simulink model "main_system312XY"  (R2020a)
settings: Solver=daessc  StartTime=0.0  StopTime=10  RelTol=1e-3
model workspace (MAT data in the model file):
  Vmax : Simulink.Parameter (value not decoded)
values from neighbouring files (symbols this model uses):
  motor_diamter = 25/1000    (= 0.025)    [parameters.m]
  motor_height = 56/1000    (= 0.056)    [parameters.m]
  pulley_diameterOut = 1/100    (= 0.01)    [parameters.m]
undefined symbols (not defined in the file or in its folder): Local, sigbuilder_block, X, Y, Z
libraries: sm_lib x59, Multibody_Parts_Lib x22, nesl_utility x7, simulink x3
(part 2 of 2)

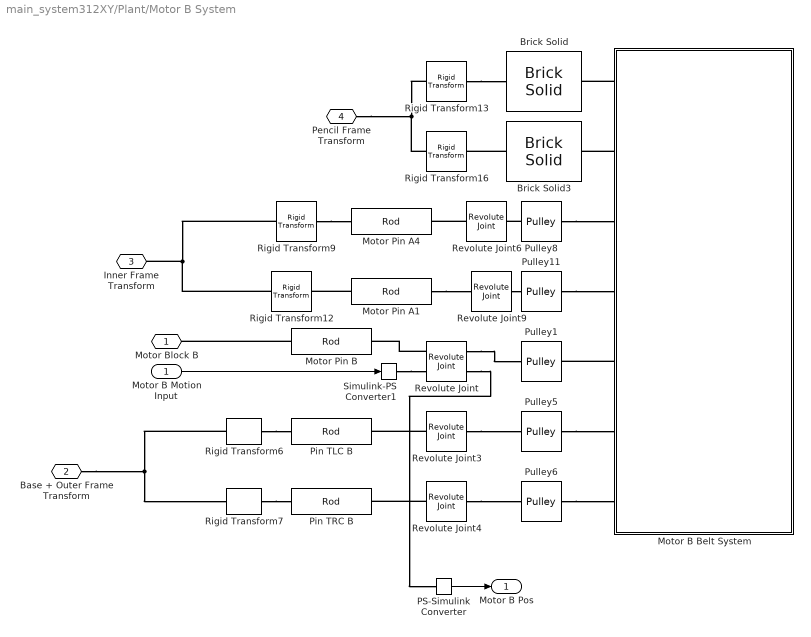
== system main_system312XY/Plant/Motor B System ==
  Motor B Motion Input : Inport
  Brick Solid : sm_lib/Body Elements/Brick Solid  GraphicAmbientColor=[0.15 0.15 0.15 1.0]  BasedOnType=Density  BrickDimensions=end_stop_size  BrickDimensionUnits=cm  CenterOfMass=[0 0 0]  CenterOfMassUnits=m  GraphicDiffuseColor=[0.5 0.5 0.5]  Density=1000  DensityUnits=kg/m^3  DoExposeReferenceFrame=on  GraphicEmissiveColor=[0.0 0.0 0.0 1.0]  ExportEntireGeometry=off  SerializedFrames=<Frames><Frame><Id>Frame1</Id><Value><Name>Bottom</Name><Origin><Source>GeometricFeature</Source><FeatureName>-z surface</FeatureName></Origin><PrimaryAxis><DefinedDirection>+Z</DefinedDirection><Source>ReferenceFrame</Source><SourceDirection>+Z</SourceDirection><FeatureName></FeatureName></PrimaryAxis><SecondaryAxis><DefinedDirection>+X</DefinedDirection><Source>ReferenceFrame</Source><SourceDirection>+X</SourceDirection><FeatureName></FeatureName></SecondaryAxis></Value></Frame></Frames>  MarkerShape=Sphere  MarkerSize=10  GraphicType=FromGeometry  InertiaType=CalculateFromGeometry  Mass=1  MassUnits=kg  MomentsOfInertia=[1 1 1]  MomentsOfInertiaUnits=kg*m^2  GraphicOpacity=1.0  ProductsOfInertia=[0 0 0]  ProductsOfInertiaUnits=kg*m^2  GraphicShininess=75  GraphicSpecularColor=[0.5 0.5 0.5 1.0]  GraphicVisPropType=SimpleVisualProperties
  Brick Solid3 : sm_lib/Body Elements/Brick Solid  GraphicAmbientColor=[0.15 0.15 0.15 1.0]  BasedOnType=Density  BrickDimensions=end_stop_size  BrickDimensionUnits=cm  CenterOfMass=[0 0 0]  CenterOfMassUnits=m  GraphicDiffuseColor=[0.5 0.5 0.5]  Density=1000  DensityUnits=kg/m^3  DoExposeReferenceFrame=on  GraphicEmissiveColor=[0.0 0.0 0.0 1.0]  ExportEntireGeometry=off  SerializedFrames=<Frames><Frame><Id>Frame1</Id><Value><Name>Bottom</Name><Origin><Source>GeometricFeature</Source><FeatureName>-z surface</FeatureName></Origin><PrimaryAxis><DefinedDirection>+Z</DefinedDirection><Source>ReferenceFrame</Source><SourceDirection>+Z</SourceDirection><FeatureName></FeatureName></PrimaryAxis><SecondaryAxis><DefinedDirection>+X</DefinedDirection><Source>ReferenceFrame</Source><SourceDirection>+X</SourceDirection><FeatureName></FeatureName></SecondaryAxis></Value></Frame></Frames>  MarkerShape=Sphere  MarkerSize=10  GraphicType=FromGeometry  InertiaType=CalculateFromGeometry  Mass=1  MassUnits=kg  MomentsOfInertia=[1 1 1]  MomentsOfInertiaUnits=kg*m^2  GraphicOpacity=1.0  ProductsOfInertia=[0 0 0]  ProductsOfInertiaUnits=kg*m^2  GraphicShininess=75  GraphicSpecularColor=[0.5 0.5 0.5 1.0]  GraphicVisPropType=SimpleVisualProperties
  Motor B Belt System : Subsystem
  Motor Pin A1 : Multibody_Parts_Lib/Basic/Rod  rod_rad=pulley_diameterInner  rod_len=pulley_pin_height  rod_rho=7000  rod_color=motor_colA  rod_opc=1  popup_zori=Local +Z  popup_markings=None  mark_radius_range=[0.5 1.01]  mark_length_range=1.005  mark_angle_range=30  mark_color=[1 1 1]
      settings: SourceProductName=Simscape Multibody Parts Library
  Motor Pin A4 : Multibody_Parts_Lib/Basic/Rod  rod_rad=pulley_diameterInner  rod_len=pulley_pin_height  rod_rho=7000  rod_color=motor_colA  rod_opc=1  popup_zori=Local +Z  popup_markings=None  mark_radius_range=[0.5 1.01]  mark_length_range=1.005  mark_angle_range=30  mark_color=[1 1 1]
      settings: SourceProductName=Simscape Multibody Parts Library
  Motor Pin B : Multibody_Parts_Lib/Basic/Rod  rod_rad=pulley_diameterInner  rod_len=pulley_pin_height  rod_rho=7000  rod_color=motor_colB  rod_opc=1  popup_zori=Local +Z  popup_markings=None  mark_radius_range=[0.5 1.01]  mark_length_range=1.005  mark_angle_range=30  mark_color=[1 1 1]
      settings: SourceProductName=Simscape Multibody Parts Library
  PS-Simulink Converter : nesl_utility/PS-Simulink Converter  PhysicalDomain=network_engine_domain  SubClassName=ps_output  LeftPortType=input  RightPortType=output  PseudoPeriodic=off  Frequencies=[]  Unit=inherit  AffineConversion=off
  Pin TLC B : Multibody_Parts_Lib/Basic/Rod  rod_rad=pulley_diameterInner  rod_len=pulley_pin_height  rod_rho=7000  rod_color=motor_colA  rod_opc=1  popup_zori=Local +Z  popup_markings=None  mark_radius_range=[0.5 1.01]  mark_length_range=1.005  mark_angle_range=30  mark_color=[1 1 1]
      settings: SourceProductName=Simscape Multibody Parts Library
  Pin TRC B : Multibody_Parts_Lib/Basic/Rod  rod_rad=pulley_diameterInner  rod_len=pulley_pin_height  rod_rho=7000  rod_color=motor_colA  rod_opc=1  popup_zori=Local +Z  popup_markings=None  mark_radius_range=[0.5 1.01]  mark_length_range=1.005  mark_angle_range=30  mark_color=[1 1 1]
      settings: SourceProductName=Simscape Multibody Parts Library
  Pulley1 : Multibody_Parts_Lib/Basic/Pulley  pulley_rad=pulley_diameterOut/2  pulley_d_grv=pulley_diameterOut/2  pulley_a_grv=45  pulley_th=pulley_height  pulley_radh=0.005  pulley_rho=7000  pulley_clr=[0.6 0.6 0.6]  pulley_opc=1  pulley_zori=No  popup_markings=Two  mark_radius_range=[0.7 0.9]  mark_angle_range=60  mark_color=[1 1 1]
      settings: SourceProductName=Simscape Multibody Parts Library
  Pulley11 : Multibody_Parts_Lib/Basic/Pulley  pulley_rad=pulley_diameterOut/2  pulley_d_grv=pulley_diameterOut/2  pulley_a_grv=45  pulley_th=0.01  pulley_radh=0.005  pulley_rho=7000  pulley_clr=[0.6 0.6 0.6]  pulley_opc=1  pulley_zori=No  popup_markings=Two  mark_radius_range=[0.7 0.9]  mark_angle_range=60  mark_color=[1 1 1]
      settings: SourceProductName=Simscape Multibody Parts Library
  Pulley5 : Multibody_Parts_Lib/Basic/Pulley  pulley_rad=pulley_diameterOut/2  pulley_d_grv=pulley_diameterOut/2  pulley_a_grv=45  pulley_th=pulley_height  pulley_radh=0.005  pulley_rho=7000  pulley_clr=[0.6 0.6 0.6]  pulley_opc=1  pulley_zori=No  popup_markings=Two  mark_radius_range=[0.7 0.9]  mark_angle_range=60  mark_color=[1 1 1]
      settings: SourceProductName=Simscape Multibody Parts Library
  Pulley6 : Multibody_Parts_Lib/Basic/Pulley  pulley_rad=pulley_diameterOut/2  pulley_d_grv=pulley_diameterOut/2  pulley_a_grv=45  pulley_th=pulley_height  pulley_radh=0.005  pulley_rho=7000  pulley_clr=[0.6 0.6 0.6]  pulley_opc=1  pulley_zori=No  popup_markings=Two  mark_radius_range=[0.7 0.9]  mark_angle_range=60  mark_color=[1 1 1]
      settings: SourceProductName=Simscape Multibody Parts Library
  Pulley8 : Multibody_Parts_Lib/Basic/Pulley  pulley_rad=pulley_diameterOut/2  pulley_d_grv=pulley_diameterOut/2  pulley_a_grv=45  pulley_th=0.01  pulley_radh=0.005  pulley_rho=7000  pulley_clr=[0.6 0.6 0.6]  pulley_opc=1  pulley_zori=No  popup_markings=Two  mark_radius_range=[0.7 0.9]  mark_angle_range=60  mark_color=[1 1 1]
      settings: SourceProductName=Simscape Multibody Parts Library
  Revolute Joint : sm_lib/Joints/Revolute Joint  JointMode=Normal  SenseConstraintForce=off  SenseConstraintForceX=off  SenseConstraintForceY=off  SenseConstraintForceZ=off  SenseConstraintTorque=off  SenseConstraintTorqueX=off  SenseConstraintTorqueY=off  SenseConstraintTorqueZ=off  SenseTotalForce=off  SenseTotalForceX=off  SenseTotalForceY=off  SenseTotalForceZ=off  SenseTotalTorque=off  SenseTotalTorqueX=off  SenseTotalTorqueY=off  SenseTotalTorqueZ=off  CompositeWrenchDir=FollowerOnBase  CompositeWrenchFrame=BaseFrame  EquilibriumPosition=0  EquilibriumPositionUnits=deg  SpringStiffness=0  SpringStiffnessUnits=N*m/deg  DampingCoefficient=0  DampingCoefficientUnits=N*m/(deg/s)  TorqueActuationMode=ComputedTorque  MotionActuationMode=InputMotion  SensePosition=on  SenseVelocity=off  SenseAcceleration=off  SenseTorqueForce=off  SenseLowerLimitTorqueForce=off  SenseUpperLimitTorqueForce=off  LowerLimitSpecify=off  LowerLimitBound=-90  LowerLimitBoundUnits=deg  LowerLimitStiffness=1e4  LowerLimitStiffnessUnits=N*m/deg  LowerLimitDamping=10  LowerLimitDampingUnits=N*m/(deg/s)  LowerLimitTransitionRegionWidth=0.1  LowerLimitTransitionRegionWidthUnits=deg  UpperLimitSpecify=off  UpperLimitBound=90  UpperLimitBoundUnits=deg  UpperLimitStiffness=1e4  UpperLimitStiffnessUnits=N*m/deg  UpperLimitDamping=10  UpperLimitDampingUnits=N*m/(deg/s)  UpperLimitTransitionRegionWidth=0.1  UpperLimitTransitionRegionWidthUnits=deg  PositionTargetSpecify=off  PositionTargetPriority=High  PositionTargetValue=0  PositionTargetValueUnits=deg  VelocityTargetSpecify=off  VelocityTargetPriority=High  VelocityTargetValue=0  VelocityTargetValueUnits=deg/s
  Revolute Joint{3..4,6,9} (4 alike) : sm_lib/Joints/Revolute Joint  JointMode=Normal  SenseConstraintForce=off  SenseConstraintForceX=off  SenseConstraintForceY=off  SenseConstraintForceZ=off  SenseConstraintTorque=off  SenseConstraintTorqueX=off  SenseConstraintTorqueY=off  SenseConstraintTorqueZ=off  SenseTotalForce=off  SenseTotalForceX=off  SenseTotalForceY=off  SenseTotalForceZ=off  SenseTotalTorque=off  SenseTotalTorqueX=off  SenseTotalTorqueY=off  SenseTotalTorqueZ=off  CompositeWrenchDir=FollowerOnBase  CompositeWrenchFrame=BaseFrame  EquilibriumPosition=0  EquilibriumPositionUnits=deg  SpringStiffness=0  SpringStiffnessUnits=N*m/deg  DampingCoefficient=0  DampingCoefficientUnits=N*m/(deg/s)  TorqueActuationMode=NoTorque  MotionActuationMode=ComputedMotion  SensePosition=off  SenseVelocity=off  SenseAcceleration=off  SenseTorqueForce=off  SenseLowerLimitTorqueForce=off  SenseUpperLimitTorqueForce=off  LowerLimitSpecify=off  LowerLimitBound=-90  LowerLimitBoundUnits=deg  LowerLimitStiffness=1e4  LowerLimitStiffnessUnits=N*m/deg  LowerLimitDamping=10  LowerLimitDampingUnits=N*m/(deg/s)  LowerLimitTransitionRegionWidth=0.1  LowerLimitTransitionRegionWidthUnits=deg  UpperLimitSpecify=off  UpperLimitBound=90  UpperLimitBoundUnits=deg  UpperLimitStiffness=1e4  UpperLimitStiffnessUnits=N*m/deg  UpperLimitDamping=10  UpperLimitDampingUnits=N*m/(deg/s)  UpperLimitTransitionRegionWidth=0.1  UpperLimitTransitionRegionWidthUnits=deg  PositionTargetSpecify=off  PositionTargetPriority=High  PositionTargetValue=0  PositionTargetValueUnits=deg  VelocityTargetSpecify=off  VelocityTargetPriority=High  VelocityTargetValue=0  VelocityTargetValueUnits=deg/s
  Rigid Transform12 : sm_lib/Frames and Transforms/Rigid Transform  TranslationMethod=Cartesian  TranslationStandardOffset=motor_height  TranslationLengthUnit=m  TranslationStandardAxis=+Z  TranslationCartesianOffset=p_ibrB  TranslationROffset=0  TranslationROffsetUnits=m  TranslationZOffset=0  TranslationZOffsetUnits=m  TranslationThetaOffset=0  TranslationThetaOffsetUnits=deg  RotationMethod=None  RotationAngleUnits=deg  RotationStandardAxis=+Z  RotationAngle=0.0  RotationArbitraryAxis=[0 0 1]  FollAlignAxisA=+X  BaseAlignAxisA=+Y  FollAlignAxisB=+Y  BaseAlignAxisB=+Z  RotationSequenceAxes=FollowerAxes  RotationSequence=XYX  RotationSequenceAngles=[0 0 0]  RotationSequenceAnglesUnits=deg  RotationMatrix=[1 0 0; 0 1 0; 0 0 1]
  Rigid Transform13 : sm_lib/Frames and Transforms/Rigid Transform  TranslationMethod=Cartesian  TranslationStandardOffset=motor_height  TranslationLengthUnit=m  TranslationStandardAxis=+Z  TranslationCartesianOffset=p_end_tlB  TranslationROffset=0  TranslationROffsetUnits=m  TranslationZOffset=0  TranslationZOffsetUnits=m  TranslationThetaOffset=0  TranslationThetaOffsetUnits=deg  RotationMethod=None  RotationAngleUnits=deg  RotationStandardAxis=+Z  RotationAngle=0.0  RotationArbitraryAxis=[0 0 1]  FollAlignAxisA=+X  BaseAlignAxisA=+Y  FollAlignAxisB=+Y  BaseAlignAxisB=+Z  RotationSequenceAxes=FollowerAxes  RotationSequence=XYX  RotationSequenceAngles=[0 0 0]  RotationSequenceAnglesUnits=deg  RotationMatrix=[1 0 0; 0 1 0; 0 0 1]
  Rigid Transform16 : sm_lib/Frames and Transforms/Rigid Transform  TranslationMethod=Cartesian  TranslationStandardOffset=motor_height  TranslationLengthUnit=m  TranslationStandardAxis=+Z  TranslationCartesianOffset=p_end_brB  TranslationROffset=0  TranslationROffsetUnits=m  TranslationZOffset=0  TranslationZOffsetUnits=m  TranslationThetaOffset=0  TranslationThetaOffsetUnits=deg  RotationMethod=None  RotationAngleUnits=deg  RotationStandardAxis=+Z  RotationAngle=0.0  RotationArbitraryAxis=[0 0 1]  FollAlignAxisA=+X  BaseAlignAxisA=+Y  FollAlignAxisB=+Y  BaseAlignAxisB=+Z  RotationSequenceAxes=FollowerAxes  RotationSequence=XYX  RotationSequenceAngles=[0 0 0]  RotationSequenceAnglesUnits=deg  RotationMatrix=[1 0 0; 0 1 0; 0 0 1]
  Rigid Transform6 : sm_lib/Frames and Transforms/Rigid Transform  TranslationMethod=Cartesian  TranslationStandardOffset=motor_height/2  TranslationLengthUnit=m  TranslationStandardAxis=+Z  TranslationCartesianOffset=p_tlcB  TranslationROffset=0  TranslationROffsetUnits=m  TranslationZOffset=0  TranslationZOffsetUnits=m  TranslationThetaOffset=0  TranslationThetaOffsetUnits=deg  RotationMethod=None  RotationAngleUnits=deg  RotationStandardAxis=+Z  RotationAngle=0.0  RotationArbitraryAxis=[0 0 1]  FollAlignAxisA=+X  BaseAlignAxisA=+Y  FollAlignAxisB=+Y  BaseAlignAxisB=+Z  RotationSequenceAxes=FollowerAxes  RotationSequence=XYX  RotationSequenceAngles=[0 0 0]  RotationSequenceAnglesUnits=deg  RotationMatrix=[1 0 0; 0 1 0; 0 0 1]
  Rigid Transform7 : sm_lib/Frames and Transforms/Rigid Transform  TranslationMethod=Cartesian  TranslationStandardOffset=motor_height/2  TranslationLengthUnit=m  TranslationStandardAxis=+Z  TranslationCartesianOffset=p_trcB  TranslationROffset=0  TranslationROffsetUnits=m  TranslationZOffset=0  TranslationZOffsetUnits=m  TranslationThetaOffset=0  TranslationThetaOffsetUnits=deg  RotationMethod=None  RotationAngleUnits=deg  RotationStandardAxis=+Z  RotationAngle=0.0  RotationArbitraryAxis=[0 0 1]  FollAlignAxisA=+X  BaseAlignAxisA=+Y  FollAlignAxisB=+Y  BaseAlignAxisB=+Z  RotationSequenceAxes=FollowerAxes  RotationSequence=XYX  RotationSequenceAngles=[0 0 0]  RotationSequenceAnglesUnits=deg  RotationMatrix=[1 0 0; 0 1 0; 0 0 1]
  Rigid Transform9 : sm_lib/Frames and Transforms/Rigid Transform  TranslationMethod=Cartesian  TranslationStandardOffset=motor_height  TranslationLengthUnit=m  TranslationStandardAxis=+Z  TranslationCartesianOffset=p_itlB  TranslationROffset=0  TranslationROffsetUnits=m  TranslationZOffset=0  TranslationZOffsetUnits=m  TranslationThetaOffset=0  TranslationThetaOffsetUnits=deg  RotationMethod=None  RotationAngleUnits=deg  RotationStandardAxis=+Z  RotationAngle=0.0  RotationArbitraryAxis=[0 0 1]  FollAlignAxisA=+X  BaseAlignAxisA=+Y  FollAlignAxisB=+Y  BaseAlignAxisB=+Z  RotationSequenceAxes=FollowerAxes  RotationSequence=XYX  RotationSequenceAngles=[0 0 0]  RotationSequenceAnglesUnits=deg  RotationMatrix=[1 0 0; 0 1 0; 0 0 1]
  Simulink-PS Converter1 : nesl_utility/Simulink-PS Converter  PhysicalDomain=network_engine_domain  SubClassName=ps_input  LeftPortType=input  RightPortType=output  PseudoPeriodic=off  Frequencies=[]  NoiseDistribution=none  NoiseParameters=[]  Unit=1  AffineConversion=off  FilteringAndDerivatives=filter  SimscapeFilterOrder=2  InputFilterTimeConstant=0.001  UdotUserProvided=0
  Motor Block B : PMIOPort  Side=Left
  Base + Outer Frame Transform : PMIOPort  Port=2  Side=Left
  Inner Frame Transform : PMIOPort  Port=3  Side=Left
  Pencil Frame Transform : PMIOPort  Port=4  Side=Left
  Motor B Pos : Outport
  wires:
  Motor B Motion Input/1 -> Simulink-PS Converter1/1
  PS-Simulink Converter/1 -> Motor B Pos/1
  connections:
  Motor Pin A1/RConn1 -- Revolute Joint9/LConn1
  Revolute Joint/LConn1 -- Motor Pin B/RConn1
  Rigid Transform16/LConn1 -- Pencil Frame Transform/RConn1 -- Rigid Transform13/LConn1
  Pulley8/RConn1 -- Revolute Joint6/RConn1
  Pulley5/RConn1 -- Motor B Belt System/LConn6
  Rigid Transform7/RConn1 -- Pin TRC B/LConn1
  Revolute Joint4/LConn1 -- Pin TRC B/RConn1
  Pulley8/LConn1 -- Motor B Belt System/LConn3
  Rigid Transform6/RConn1 -- Pin TLC B/LConn1
  Rigid Transform6/LConn1 -- Base + Outer Frame Transform/RConn1 -- Rigid Transform7/LConn1
  Motor B Belt System/LConn1 -- Brick Solid/RConn1
  Revolute Joint/RConn1 -- Pulley1/LConn1
  Rigid Transform9/RConn1 -- Motor Pin A4/LConn1
  Revolute Joint6/LConn1 -- Motor Pin A4/RConn1
  Revolute Joint4/RConn1 -- Pulley6/LConn1
  Rigid Transform9/LConn1 -- Inner Frame Transform/RConn1 -- Rigid Transform12/LConn1
  Pulley11/LConn1 -- Motor B Belt System/LConn4
  Rigid Transform13/RConn1 -- Brick Solid/LConn1
  Motor Pin B/LConn1 -- Motor Block B/RConn1
  Revolute Joint3/LConn1 -- Pin TLC B/RConn1
  Revolute Joint3/RConn1 -- Pulley5/LConn1
  Brick Solid3/LConn1 -- Rigid Transform16/RConn1
  Pulley6/RConn1 -- Motor B Belt System/LConn7
  Motor B Belt System/LConn2 -- Brick Solid3/RConn1
  Motor B Belt System/LConn5 -- Pulley1/RConn1
  Motor Pin A1/LConn1 -- Rigid Transform12/RConn1
  Revolute Joint9/RConn1 -- Pulley11/RConn1
  Simulink-PS Converter1/RConn1 -- Revolute Joint/LConn2
  Revolute Joint/RConn2 -- PS-Simulink Converter/LConn1

== system main_system312XY/Plant/Motor Height Transform ==
  Rigid Transform4 : sm_lib/Frames and Transforms/Rigid Transform  TranslationMethod=StandardAxis  TranslationStandardOffset=motor_height  TranslationLengthUnit=m  TranslationStandardAxis=+Z  TranslationCartesianOffset=[0 0 0]  TranslationROffset=0  TranslationROffsetUnits=m  TranslationZOffset=0  TranslationZOffsetUnits=m  TranslationThetaOffset=0  TranslationThetaOffsetUnits=deg  RotationMethod=None  RotationAngleUnits=deg  RotationStandardAxis=+Z  RotationAngle=0.0  RotationArbitraryAxis=[0 0 1]  FollAlignAxisA=+X  BaseAlignAxisA=+Y  FollAlignAxisB=+Y  BaseAlignAxisB=+Z  RotationSequenceAxes=FollowerAxes  RotationSequence=XYX  RotationSequenceAngles=[0 0 0]  RotationSequenceAnglesUnits=deg  RotationMatrix=[1 0 0; 0 1 0; 0 0 1]
  B : PMIOPort  Side=Right
  F : PMIOPort  Port=2  Side=Left
  connections:
  Rigid Transform4/RConn1 -- B/RConn1
  Rigid Transform4/LConn1 -- F/RConn1

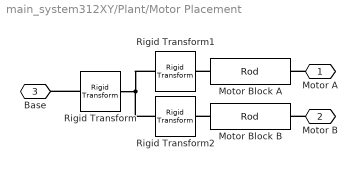
== system main_system312XY/Plant/Motor Placement ==
  Motor Block A : Multibody_Parts_Lib/Basic/Rod  rod_rad=motor_diamter/2  rod_len=motor_height  rod_rho=7000  rod_color=motor_colA  rod_opc=1  popup_zori=Local +Z  popup_markings=None  mark_radius_range=[0.5 1.01]  mark_length_range=1.005  mark_angle_range=30  mark_color=[1 1 1]
      settings: SourceProductName=Simscape Multibody Parts Library
  Motor Block B : Multibody_Parts_Lib/Basic/Rod  rod_rad=motor_diamter/2  rod_len=motor_height  rod_rho=7000  rod_color=motor_colB  rod_opc=1  popup_zori=Local +Z  popup_markings=None  mark_radius_range=[0.5 1.01]  mark_length_range=1.005  mark_angle_range=30  mark_color=[1 1 1]
      settings: SourceProductName=Simscape Multibody Parts Library
  Rigid Transform : sm_lib/Frames and Transforms/Rigid Transform  TranslationMethod=StandardAxis  TranslationStandardOffset=motorDisplacement_y  TranslationLengthUnit=m  TranslationStandardAxis=-Y  TranslationCartesianOffset=[0 0 0]  TranslationROffset=0  TranslationROffsetUnits=m  TranslationZOffset=0  TranslationZOffsetUnits=m  TranslationThetaOffset=0  TranslationThetaOffsetUnits=deg  RotationMethod=None  RotationAngleUnits=deg  RotationStandardAxis=+Z  RotationAngle=0.0  RotationArbitraryAxis=[0 0 1]  FollAlignAxisA=+X  BaseAlignAxisA=+Y  FollAlignAxisB=+Y  BaseAlignAxisB=+Z  RotationSequenceAxes=FollowerAxes  RotationSequence=XYX  RotationSequenceAngles=[0 0 0]  RotationSequenceAnglesUnits=deg  RotationMatrix=[1 0 0; 0 1 0; 0 0 1]
  Rigid Transform1 : sm_lib/Frames and Transforms/Rigid Transform  TranslationMethod=StandardAxis  TranslationStandardOffset=motorDisplacement_x  TranslationLengthUnit=m  TranslationStandardAxis=-X  TranslationCartesianOffset=[0 0 0]  TranslationROffset=0  TranslationROffsetUnits=m  TranslationZOffset=0  TranslationZOffsetUnits=m  TranslationThetaOffset=0  TranslationThetaOffsetUnits=deg  RotationMethod=StandardAxis  RotationAngleUnits=deg  RotationStandardAxis=-X  RotationAngle=0.0  RotationArbitraryAxis=[0 0 1]  FollAlignAxisA=+X  BaseAlignAxisA=+Y  FollAlignAxisB=+Y  BaseAlignAxisB=+Z  RotationSequenceAxes=FollowerAxes  RotationSequence=XYX  RotationSequenceAngles=[0 0 0]  RotationSequenceAnglesUnits=deg  RotationMatrix=[1 0 0; 0 1 0; 0 0 1]
  Rigid Transform2 : sm_lib/Frames and Transforms/Rigid Transform  TranslationMethod=StandardAxis  TranslationStandardOffset=motorDisplacement_x  TranslationLengthUnit=m  TranslationStandardAxis=+X  TranslationCartesianOffset=[0 0 0]  TranslationROffset=0  TranslationROffsetUnits=m  TranslationZOffset=0  TranslationZOffsetUnits=m  TranslationThetaOffset=0  TranslationThetaOffsetUnits=deg  RotationMethod=StandardAxis  RotationAngleUnits=deg  RotationStandardAxis=-X  RotationAngle=0.0  RotationArbitraryAxis=[0 0 1]  FollAlignAxisA=+X  BaseAlignAxisA=+Y  FollAlignAxisB=+Y  BaseAlignAxisB=+Z  RotationSequenceAxes=FollowerAxes  RotationSequence=XYX  RotationSequenceAngles=[0 0 0]  RotationSequenceAnglesUnits=deg  RotationMatrix=[1 0 0; 0 1 0; 0 0 1]
  Motor A : PMIOPort  Side=Right
  Motor B : PMIOPort  Port=2  Side=Right
  Base : PMIOPort  Port=3  Side=Left
  connections:
  Motor Block A/LConn1 -- Rigid Transform1/RConn1
  Motor B/RConn1 -- Motor Block B/RConn1
  Rigid Transform1/LConn1 -- Rigid Transform/RConn1 -- Rigid Transform2/LConn1
  Motor A/RConn1 -- Motor Block A/RConn1
  Rigid Transform/LConn1 -- Base/RConn1
  Motor Block B/LConn1 -- Rigid Transform2/RConn1

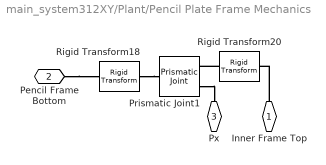
== system main_system312XY/Plant/Pencil Plate Frame Mechanics ==
  Prismatic Joint1 : sm_lib/Joints/Prismatic Joint  JointMode=Normal  SenseConstraintForce=off  SenseConstraintForceX=off  SenseConstraintForceY=off  SenseConstraintForceZ=off  SenseConstraintTorque=off  SenseConstraintTorqueX=off  SenseConstraintTorqueY=off  SenseConstraintTorqueZ=off  SenseTotalForce=off  SenseTotalForceX=off  SenseTotalForceY=off  SenseTotalForceZ=off  SenseTotalTorque=off  SenseTotalTorqueX=off  SenseTotalTorqueY=off  SenseTotalTorqueZ=off  CompositeWrenchDir=FollowerOnBase  CompositeWrenchFrame=BaseFrame  EquilibriumPosition=0  EquilibriumPositionUnits=m  SpringStiffness=0  SpringStiffnessUnits=N/m  DampingCoefficient=0  DampingCoefficientUnits=N/(m/s)  TorqueActuationMode=NoTorque  MotionActuationMode=ComputedMotion  SensePosition=on  SenseVelocity=off  SenseAcceleration=off  SenseTorqueForce=off  SenseLowerLimitTorqueForce=off  SenseUpperLimitTorqueForce=off  LowerLimitSpecify=on  LowerLimitBound=-0.15  LowerLimitBoundUnits=m  LowerLimitStiffness=1e6  LowerLimitStiffnessUnits=N/m  LowerLimitDamping=1e3  LowerLimitDampingUnits=N/(m/s)  LowerLimitTransitionRegionWidth=1e-4  LowerLimitTransitionRegionWidthUnits=m  UpperLimitSpecify=on  UpperLimitBound=0.15  UpperLimitBoundUnits=m  UpperLimitStiffness=1e6  UpperLimitStiffnessUnits=N/m  UpperLimitDamping=1e3  UpperLimitDampingUnits=N/(m/s)  UpperLimitTransitionRegionWidth=1e-4  UpperLimitTransitionRegionWidthUnits=m  PositionTargetSpecify=off  PositionTargetPriority=High  PositionTargetValue=0  PositionTargetValueUnits=m  VelocityTargetSpecify=off  VelocityTargetPriority=High  VelocityTargetValue=0  VelocityTargetValueUnits=m/s
  Rigid Transform18 : sm_lib/Frames and Transforms/Rigid Transform  TranslationMethod=None  TranslationStandardOffset=0.1  TranslationLengthUnit=m  TranslationStandardAxis=+Z  TranslationCartesianOffset=p_itlB  TranslationROffset=0  TranslationROffsetUnits=m  TranslationZOffset=0  TranslationZOffsetUnits=m  TranslationThetaOffset=0  TranslationThetaOffsetUnits=deg  RotationMethod=StandardAxis  RotationAngleUnits=deg  RotationStandardAxis=-Y  RotationAngle=90  RotationArbitraryAxis=[0 0 1]  FollAlignAxisA=+X  BaseAlignAxisA=+Y  FollAlignAxisB=+Y  BaseAlignAxisB=+Z  RotationSequenceAxes=FollowerAxes  RotationSequence=XYX  RotationSequenceAngles=[0 0 0]  RotationSequenceAnglesUnits=deg  RotationMatrix=[1 0 0; 0 1 0; 0 0 1]
  Rigid Transform20 : sm_lib/Frames and Transforms/Rigid Transform  TranslationMethod=None  TranslationStandardOffset=0.1  TranslationLengthUnit=m  TranslationStandardAxis=-Z  TranslationCartesianOffset=p_itlB  TranslationROffset=0  TranslationROffsetUnits=m  TranslationZOffset=0  TranslationZOffsetUnits=m  TranslationThetaOffset=0  TranslationThetaOffsetUnits=deg  RotationMethod=StandardAxis  RotationAngleUnits=deg  RotationStandardAxis=+Y  RotationAngle=90  RotationArbitraryAxis=[0 0 1]  FollAlignAxisA=+X  BaseAlignAxisA=+Y  FollAlignAxisB=+Y  BaseAlignAxisB=+Z  RotationSequenceAxes=FollowerAxes  RotationSequence=XYX  RotationSequenceAngles=[0 0 0]  RotationSequenceAnglesUnits=deg  RotationMatrix=[1 0 0; 0 1 0; 0 0 1]
  Inner Frame Top : PMIOPort  Side=Right
  Pencil Frame Bottom : PMIOPort  Port=2  Side=Right
  Px : PMIOPort  Port=3  Side=Right
  connections:
  Rigid Transform18/RConn1 -- Prismatic Joint1/LConn1
  Rigid Transform20/LConn1 -- Prismatic Joint1/RConn1
  Prismatic Joint1/RConn2 -- Px/RConn1
  Inner Frame Top/RConn1 -- Rigid Transform20/RConn1
  Pencil Frame Bottom/RConn1 -- Rigid Transform18/LConn1

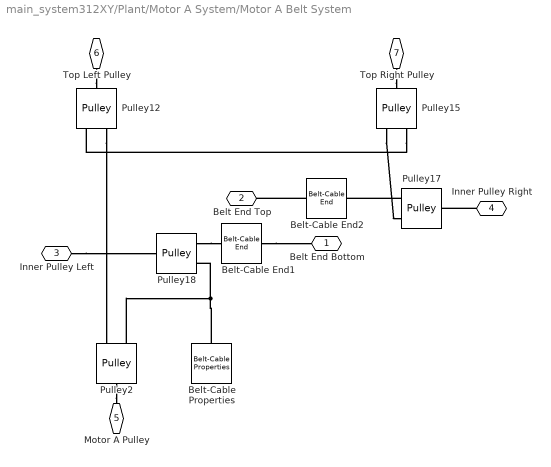
== system main_system312XY/Plant/Motor A System/Motor A Belt System ==
  Belt-Cable Properties : sm_lib/Belts and Cables/Belt-Cable Properties  DrumBeltCableAlignment=MonitoredPlanar  GraphicType=PitchLine  GraphicVisPropType=SimpleVisualProperties  GraphicDiffuseColor=motor_colA  GraphicSpecularColor=[0.5 0.5 0.5 1.0]  GraphicAmbientColor=[0.15 0.15 0.15 1.0]  GraphicEmissiveColor=[0.0 0.0 0.0 1.0]  GraphicShininess=75  GraphicOpacity=1.0
      settings: SourceProductBaseCode=MS
  Belt-Cable End1 : sm_lib/Belts and Cables/Belt-Cable End
      settings: SourceProductBaseCode=MS
  Belt-Cable End2 : sm_lib/Belts and Cables/Belt-Cable End
      settings: SourceProductBaseCode=MS
  Pulley{2,12,15,17..18} (5 alike) : sm_lib/Belts and Cables/Pulley  PitchRadius=5  PitchRadiusUnits=mm  InitialWrapAngleLowerBound=0.0  InitialWrapAngleLowerBoundUnits=deg  SenseWrapAngle=off  SensePulleyAngleA=off  SensePulleyAngleB=off  SenseFleetAngleA=off  SenseFleetAngleB=off
      settings: SourceProductBaseCode=MS
  Belt End Bottom : PMIOPort  Side=Left
  Belt End Top : PMIOPort  Port=2  Side=Left
  Inner Pulley Left : PMIOPort  Port=3  Side=Left
  Inner Pulley Right : PMIOPort  Port=4  Side=Left
  Motor A Pulley : PMIOPort  Port=5  Side=Left
  Top Left Pulley : PMIOPort  Port=6  Side=Left
  Top Right Pulley : PMIOPort  Port=7  Side=Left
  connections:
  Pulley18/RConn1 -- Belt-Cable End1/RConn1
  Belt-Cable Properties/LConn1 -- Pulley2/RConn2 -- Pulley18/RConn2
  Top Right Pulley/RConn1 -- Pulley15/LConn1
  Pulley15/RConn2 -- Pulley12/RConn1
  Pulley2/LConn1 -- Motor A Pulley/RConn1
  Top Left Pulley/RConn1 -- Pulley12/LConn1
  Belt-Cable End2/LConn1 -- Belt End Top/RConn1
  Belt-Cable End1/LConn1 -- Belt End Bottom/RConn1
  Inner Pulley Right/RConn1 -- Pulley17/LConn1
  Inner Pulley Left/RConn1 -- Pulley18/LConn1
  Pulley15/RConn1 -- Pulley17/RConn2
  Pulley17/RConn1 -- Belt-Cable End2/RConn1
  Pulley12/RConn2 -- Pulley2/RConn1

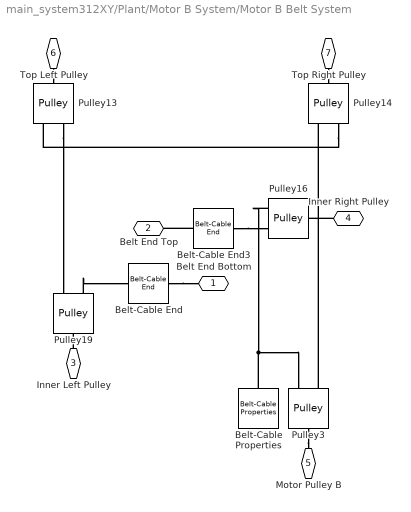
== system main_system312XY/Plant/Motor B System/Motor B Belt System ==
  Belt-Cable Properties : sm_lib/Belts and Cables/Belt-Cable Properties  DrumBeltCableAlignment=Unrestricted  GraphicType=PitchLine  GraphicVisPropType=SimpleVisualProperties  GraphicDiffuseColor=motor_colB  GraphicSpecularColor=[0.5 0.5 0.5 1.0]  GraphicAmbientColor=[0.15 0.15 0.15 1.0]  GraphicEmissiveColor=[0.0 0.0 0.0 1.0]  GraphicShininess=75  GraphicOpacity=1.0
      settings: SourceProductBaseCode=MS
  Belt-Cable End : sm_lib/Belts and Cables/Belt-Cable End
      settings: SourceProductBaseCode=MS
  Belt-Cable End3 : sm_lib/Belts and Cables/Belt-Cable End
      settings: SourceProductBaseCode=MS
  Pulley{3,13..14,16,19} (5 alike) : sm_lib/Belts and Cables/Pulley  PitchRadius=5  PitchRadiusUnits=mm  InitialWrapAngleLowerBound=0.0  InitialWrapAngleLowerBoundUnits=deg  SenseWrapAngle=off  SensePulleyAngleA=off  SensePulleyAngleB=off  SenseFleetAngleA=off  SenseFleetAngleB=off
      settings: SourceProductBaseCode=MS
  Belt End Bottom : PMIOPort  Side=Left
  Belt End Top : PMIOPort  Port=2  Side=Left
  Inner Left Pulley : PMIOPort  Port=3  Side=Left
  Inner Right Pulley : PMIOPort  Port=4  Side=Left
  Motor Pulley B : PMIOPort  Port=5  Side=Left
  Top Left Pulley : PMIOPort  Port=6  Side=Left
  Top Right Pulley : PMIOPort  Port=7  Side=Left
  connections:
  Inner Right Pulley/RConn1 -- Pulley16/LConn1
  Pulley19/RConn2 -- Belt-Cable End/RConn1
  Pulley14/RConn2 -- Pulley13/RConn1
  Pulley3/LConn1 -- Motor Pulley B/RConn1
  Pulley3/RConn2 -- Pulley14/RConn1
  Belt-Cable Properties/LConn1 -- Pulley3/RConn1 -- Pulley16/RConn1
  Belt-Cable End/LConn1 -- Belt End Bottom/RConn1
  Pulley13/RConn2 -- Pulley19/RConn1
  Inner Left Pulley/RConn1 -- Pulley19/LConn1
  Belt-Cable End3/LConn1 -- Belt End Top/RConn1
  Top Right Pulley/RConn1 -- Pulley14/LConn1
  Top Left Pulley/RConn1 -- Pulley13/LConn1
  Belt-Cable End3/RConn1 -- Pulley16/RConn2

== matlab function main_system312XY/Saturation1 ==
  data: in input; out output; Vmax input
function out = fcn(in, Vmax)
    if in > Vmax
        in = Vmax;
    elseif in < -Vmax
        in = -Vmax;
    end
out = in;

== matlab function main_system312XY/Saturation ==
  data: in input; out output; Vmax input
function out = fcn(in, Vmax)
    if in > Vmax
        in = Vmax;
    elseif in < -Vmax
        in = -Vmax;
    end
out = in;

== matlab function main_system312XY/Coordinate Translation ==
  data: Xref input; Aref output; Yref input; Bref output; Mrad input
function [Aref, Bref] = fcn(Xref, Yref, Mrad)
    % Converts X, Y (mm) Values to motor A, B values (radians)
    % Xref mm, Yref mm, Mrad mm
    % Aref radians, Bref radians
    Aref = Mrad * (Xref + Yref) / (2 * 1000);
    Bref = Mrad * (Xref - Yref) / (2 * 1000);
end

== stateflow chart main_system312XY/State Transition Table ==
  state On
  state Saftey
  (default) -> On
  On -> Saftey : [u == 1]
      | {Vmax = 6}
  Saftey -> On : [x > 120]
      | {Vmax = 2}
  data: Vmax output; u input; x input; y input
